simulink model "SCR_Injector_ON_Off"  (R2019a)
settings: Solver=FixedStepAuto  StartTime=0.0  StopTime=100  FixedStep=0.1  RelTol=1e-3
libraries: simulink x4
settings Model: DataDictionary=SCR_Injector_ON_Off_DD.sldd  Creator=Kore  LastModifiedBy=Kore
settings ConfigComp: DVModelCoverageObjectives=MCDC  DVTestSuiteOptimization=Auto  DVDetectDeadLogic=on  DVDetectActiveLogic=on  DVDetectOutOfBounds=on  DVSaveHarnessModel=on  DVSaveReport=on  DVRebuildModelRepresentation=Always

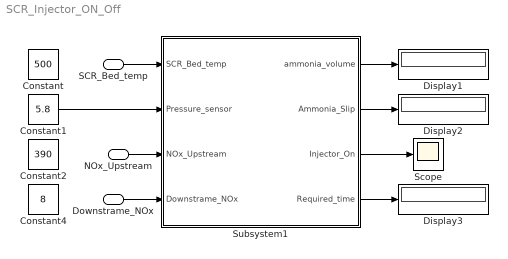
== system SCR_Injector_ON_Off ==
  NOx_Upstream : Inport
  Downstrame_NOx : Inport  Port=2
  SCR_Bed_temp : Inport  Port=3
  Constant : Constant  Value=500
  Constant1 : Constant  Value=5.8
  Constant2 : Constant  Value=390
  Constant4 : Constant  Value=8
  Display1 : Display
  Display2 : Display
  Display3 : Display
  Scope : Scope
  Subsystem1 : Subsystem
  wires:
  Subsystem1/2(Ammonia_Slip) -> Display2/1
  Subsystem1/1(ammonia_volume) -> Display1/1
  Subsystem1/3(Injector_On) -> Scope/1
  Subsystem1/4(Required_time) -> Display3/1
  Downstrame_NOx/1 -> Subsystem1/4(Downstrame_NOx)
  NOx_Upstream/1 -> Subsystem1/3(NOx_Upstream)
  SCR_Bed_temp/1 -> Subsystem1/1(SCR_Bed_temp)
  Constant1/1 -> Subsystem1/2(Pressure_sensor)

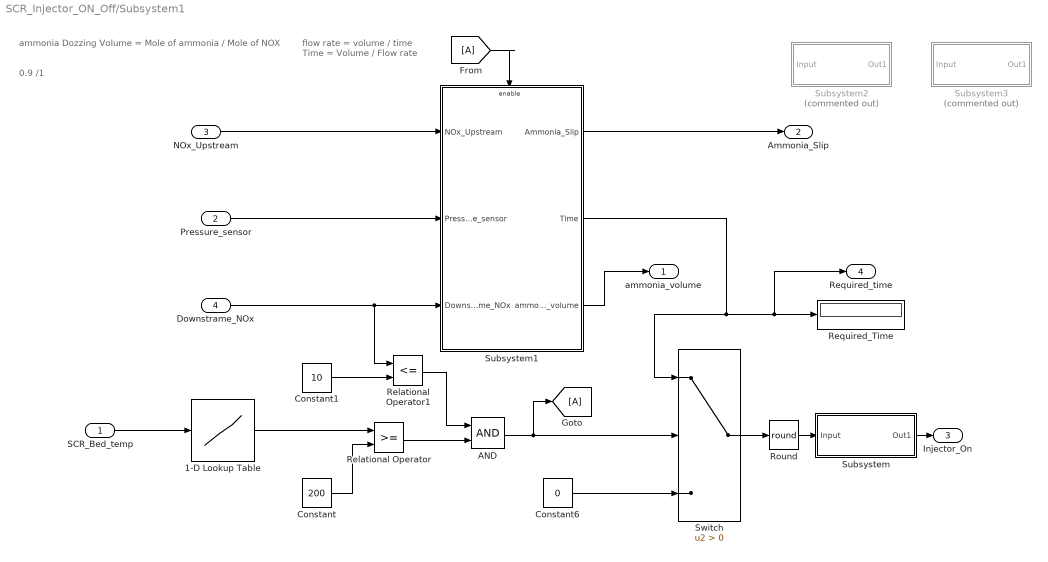
== system SCR_Injector_ON_Off/Subsystem1 ==
  note: 0.9 /1
  note: ammonia Dozzing Volume = Mole of ammonia / Mole of NOX
  note: flow rate = volume / time
      |
      | Time = Volume / Flow rate
  SCR_Bed_temp : Inport
  Pressure_sensor : Inport  Port=2
  NOx_Upstream : Inport  Port=3
  Downstrame_NOx : Inport  Port=4
  1-D Lookup Table : Lookup_n-D  NumberOfTableDimensions=1  BreakpointsForDimension1=[1:10:650]  BreakpointsForDimension2=[1:1:500]  Table=[1:10:650]  InternalRulePriority=Speed  RndMeth=Simplest  InputSameDT=on
  AND : Logic  AllPortsSameDT=off  OutDataTypeStr=boolean
  Constant : Constant  Value=200
  Constant1 : Constant  Value=10
  Constant6 : Constant  Value=0
  Relational Operator : RelationalOperator  OutDataTypeStr=boolean  RndMeth=Simplest
  Relational Operator1 : RelationalOperator  Operator=<=  OutDataTypeStr=boolean  RndMeth=Simplest
  Required_Time : Display
  Round : Rounding  Operator=round
  Subsystem : Subsystem
  Subsystem1 : Subsystem
  Subsystem2 : Subsystem  Commented=on
  Subsystem3 : Subsystem  Commented=on
  Switch : Switch  Criteria=u2 > Threshold
  ammonia_volume : Outport
  Ammonia_Slip : Outport  Port=2
  Injector_On : Outport  Port=3
  Required_time : Outport  Port=4
  wires:
  Constant/1 -> Relational Operator/2
  SCR_Bed_temp/1 -> 1-D Lookup Table/1
  1-D Lookup Table/1 -> Relational Operator/1
  Constant6/1 -> Switch/3
  Switch/1 -> Round/1
  Subsystem1/2(Time) -> Switch/1, Required_time/1, Required_Time/1
  NOx_Upstream/1 -> Subsystem1/1(NOx_Upstream)
  Pressure_sensor/1 -> Subsystem1/2(Pressure_sensor)
  Subsystem1/1(Ammonia_Slip) -> Ammonia_Slip/1
  Downstrame_NOx/1 -> Relational Operator1/1, Subsystem1/3(Downstrame_NOx)
  [A] -> Subsystem1/Enable
  Subsystem/1(Out1) -> Injector_On/1
  Round/1 -> Subsystem/1(Input)
  Relational Operator/1 -> AND/2
  AND/1 -> [A], Switch/2
  Relational Operator1/1 -> AND/1
  Constant1/1 -> Relational Operator1/2
  Subsystem1/3(ammonia_volume) -> ammonia_volume/1

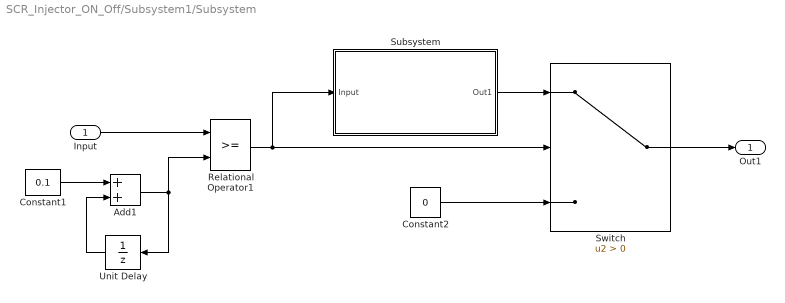
== system SCR_Injector_ON_Off/Subsystem1/Subsystem ==
  Input : Inport
  Add1 : Sum
  Constant1 : Constant  Value=0.1
  Constant2 : Constant  Value=0
  Relational Operator1 : RelationalOperator  OutDataTypeStr=boolean  RndMeth=Simplest
  Subsystem : Subsystem
  Switch : Switch  Criteria=u2 > Threshold
  Unit Delay : UnitDelay  SampleTime=-1  HasFrameUpgradeWarning=on
  Out1 : Outport
  wires:
  Constant2/1 -> Switch/3
  Unit Delay/1 -> Add1/2
  Constant1/1 -> Add1/1
  Add1/1 -> Unit Delay/1, Relational Operator1/2
  Subsystem/1(Out1) -> Switch/1
  Input/1 -> Relational Operator1/1
  Switch/1 -> Out1/1
  Relational Operator1/1 -> Switch/2, Subsystem/1(Input)

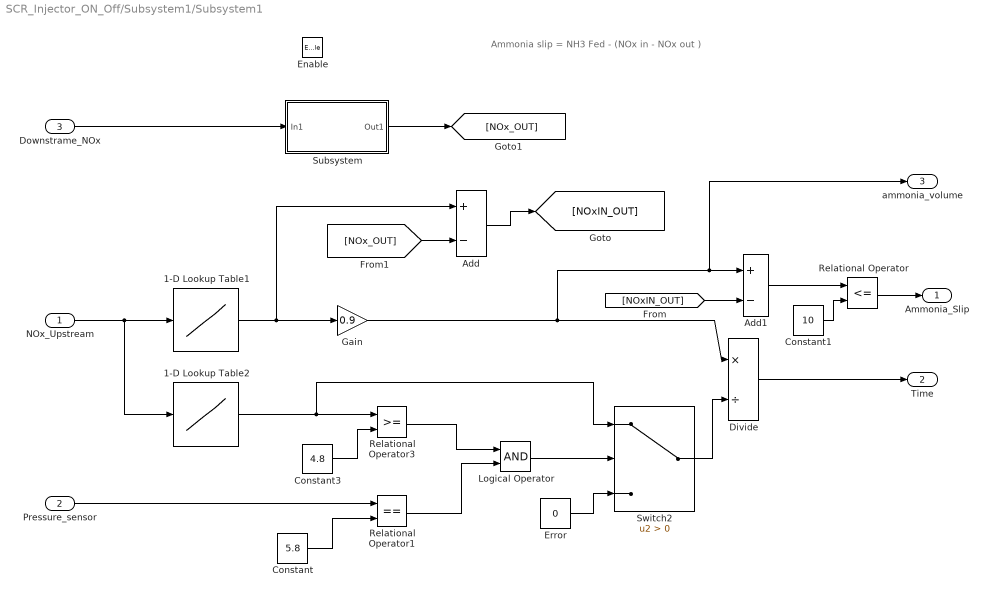
== system SCR_Injector_ON_Off/Subsystem1/Subsystem1 ==
  note: Ammonia slip = NH3 Fed - (NOx in - NOx out )
  NOx_Upstream : Inport
  Pressure_sensor : Inport  Port=2
  Downstrame_NOx : Inport  Port=3
  Enable : EnablePort  StatesWhenEnabling=reset
  1-D Lookup Table1 : Lookup_n-D  NumberOfTableDimensions=1  BreakpointsForDimension1=[1:5:650]  BreakpointsForDimension2=[1:1:500]  Table=[1:5:650]  InternalRulePriority=Speed  RndMeth=Simplest  InputSameDT=on
  1-D Lookup Table2 : Lookup_n-D  NumberOfTableDimensions=1  BreakpointsForDimension1=|  BreakpointsForDimension2=[1:1:500]  Table=|  InternalRulePriority=Speed  RndMeth=Simplest  InputSameDT=on
      BreakpointsForDimension1=|
      | [10
      | 70
      | 77.6
      | 80.4
      | 86.4
      | 99.6
      | 108
      | 117.6
      | 127.2
      | 136.8
      | 149.3
      | 158.3
      | 163.3
      | 168.3
      | 175.3
      | 181.5
      | 187.7
      | 193.9
      | 200.1
      | 206.3
      | 212.85
      | 223.5
      | 233.15
      | 242.8
      | 255.45
      | 264.9
      | 275.35
      | 285.8
      | 296.25
      | 306.7
      | 317.15
      | 327.6
      | 338.05
      | 348.5
      | 358.95
      | 369.4
      | 379.85
      | 390.3
      | 400.75
      | 411.2
      | 421.65
      | 432.1
      | 442.55
      | 453
      | 463.45
      | 473.9
      | 484.35
      | 494.8
      | 505.25
      | 515.7
      | 526.15
      | 536.6
      | 547.05
      | 557.5]
      Table=|
      | [4
      | 4
      | 4
      | 4
      | 4
      | 4
      | 4
      | 4
      | 4
      | 4.8
      | 4.8
      | 4.8
      | 4.8
      | 4.8
      | 4.8
      | 4.8
      | 4.8
      | 4.8
      | 4.8
      | 4.8
      | 4.8
      | 5.8
      | 6.4
      | 7.3
      | 8.1
      | 8.9
      | 9.7
      | 10.5
      | 11.3
      | 12.1
      | 12.9
      | 13.7
      | 14.5
      | 15.3
      | 16.1
      | 16.9
      | 17.7
      | 18.5
      | 19.3
      | 20.1
      | 20.9
      | 21.7
      | 22.5
      | 23.3
      | 24.1
      | 24.9
      | 25.7
      | 26.5
      | 27.3
      | 28.1
      | 28.9
      | 29.7
      | 30.0
      | 30.0
      | ]
  Add : Sum  Inputs=+-
  Add1 : Sum  Inputs=+-
  Constant : Constant  Value=5.8
  Constant1 : Constant  Value=10
  Constant3 : Constant  Value=4.8
  Divide : Product  Inputs=*/
  Error : Constant  Value=0
  Gain : Gain  Gain=0.9
  Logical Operator : Logic  AllPortsSameDT=off  OutDataTypeStr=boolean
  Relational Operator : RelationalOperator  Operator=<=  OutDataTypeStr=boolean  RndMeth=Simplest
  Relational Operator1 : RelationalOperator  Operator===  OutDataTypeStr=boolean  RndMeth=Simplest
  Relational Operator3 : RelationalOperator  OutDataTypeStr=boolean  RndMeth=Simplest
  Subsystem : Subsystem
  Switch2 : Switch  Criteria=u2 > Threshold
  Ammonia_Slip : Outport
  Time : Outport  Port=2
  ammonia_volume : Outport  Port=3
  wires:
  Pressure_sensor/1 -> Relational Operator1/1
  Add/1 -> [NOxIN_OUT]
  [NOx_OUT] -> Add/2
  Relational Operator1/1 -> Logical Operator/2
  Constant/1 -> Relational Operator1/2
  1-D Lookup Table1/1 -> Gain/1, Add/1
  Divide/1 -> Time/1
  Constant3/1 -> Relational Operator3/2
  Relational Operator3/1 -> Logical Operator/1
  Error/1 -> Switch2/3
  Switch2/1 -> Divide/2
  Logical Operator/1 -> Switch2/2
  [NOxIN_OUT] -> Add1/2
  Add1/1 -> Relational Operator/1
  Subsystem/1(Out1) -> [NOx_OUT]
  Downstrame_NOx/1 -> Subsystem/1(In1)
  1-D Lookup Table2/1 -> Switch2/1, Relational Operator3/1
  NOx_Upstream/1 -> 1-D Lookup Table2/1, 1-D Lookup Table1/1
  Constant1/1 -> Relational Operator/2
  Relational Operator/1 -> Ammonia_Slip/1
  Gain/1 -> Divide/1, ammonia_volume/1, Add1/1

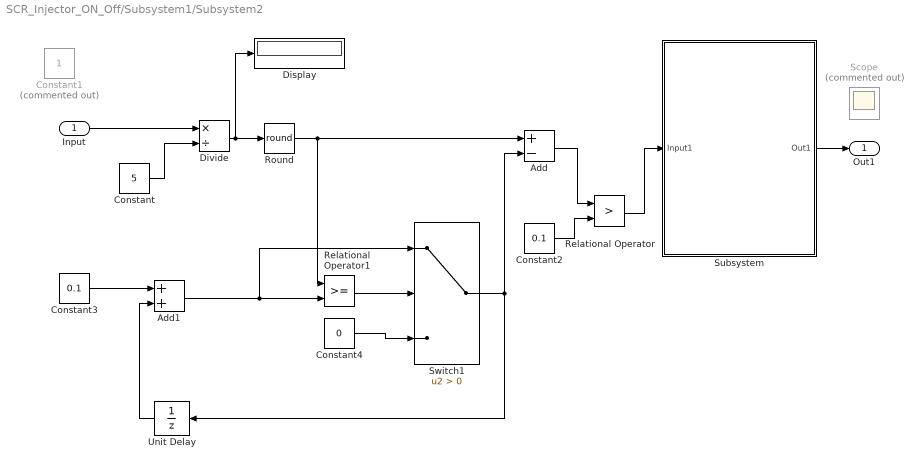
== system SCR_Injector_ON_Off/Subsystem1/Subsystem2 ==
  Input : Inport
  Add : Sum  Inputs=+-
  Add1 : Sum
  Constant : Constant  Value=5
  Constant1 : Constant  Commented=on
  Constant2 : Constant  Value=0.1
  Constant3 : Constant  Value=0.1
  Constant4 : Constant  Value=0
  Display : Display
  Divide : Product  Inputs=*/
  Relational Operator : RelationalOperator  Operator=>  OutDataTypeStr=boolean  RndMeth=Simplest
  Relational Operator1 : RelationalOperator  OutDataTypeStr=boolean  RndMeth=Simplest
  Round : Rounding  Operator=round
  Scope : Scope  Commented=on
  Subsystem : Subsystem
  Switch1 : Switch  Criteria=u2 > Threshold
  Unit Delay : UnitDelay  SampleTime=-1  HasFrameUpgradeWarning=on
  Out1 : Outport
  wires:
  Constant/1 -> Divide/2
  Divide/1 -> Round/1, Display/1
  Input/1 -> Divide/1
  Round/1 -> Relational Operator1/1, Add/1
  Constant4/1 -> Switch1/3
  Switch1/1 -> Add/2, Unit Delay/1
  Constant3/1 -> Add1/1
  Relational Operator1/1 -> Switch1/2
  Add1/1 -> Switch1/1, Relational Operator1/2
  Unit Delay/1 -> Add1/2
  Subsystem/1(Out1) -> Out1/1
  Add/1 -> Relational Operator/1
  Relational Operator/1 -> Subsystem/1(Input1)
  Constant2/1 -> Relational Operator/2

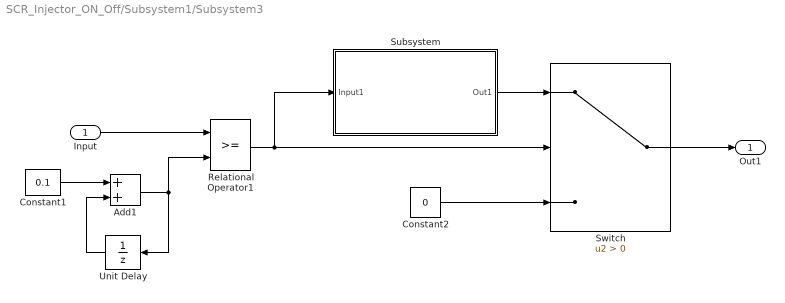
== system SCR_Injector_ON_Off/Subsystem1/Subsystem3 ==
  Input : Inport
  Add1 : Sum
  Constant1 : Constant  Value=0.1
  Constant2 : Constant  Value=0
  Relational Operator1 : RelationalOperator  OutDataTypeStr=boolean  RndMeth=Simplest
  Subsystem : Subsystem
  Switch : Switch  Criteria=u2 > Threshold
  Unit Delay : UnitDelay  SampleTime=-1  HasFrameUpgradeWarning=on
  Out1 : Outport
  wires:
  Relational Operator1/1 -> Switch/2, Subsystem/1(Input1)
  Switch/1 -> Out1/1
  Input/1 -> Relational Operator1/1
  Subsystem/1(Out1) -> Switch/1
  Add1/1 -> Relational Operator1/2, Unit Delay/1
  Constant1/1 -> Add1/1
  Unit Delay/1 -> Add1/2
  Constant2/1 -> Switch/3

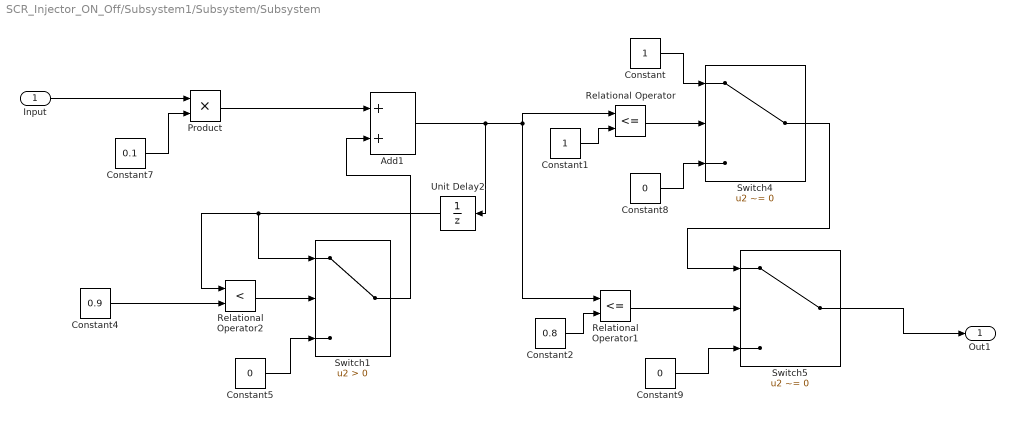
== system SCR_Injector_ON_Off/Subsystem1/Subsystem/Subsystem ==
  Input : Inport
  Add1 : Sum
  Constant : Constant
  Constant1 : Constant
  Constant2 : Constant  Value=0.8
  Constant4 : Constant  Value=0.9
  Constant5 : Constant  Value=0
  Constant7 : Constant  Value=0.1
  Constant8 : Constant  Value=0
  Constant9 : Constant  Value=0
  Product : Product
  Relational Operator : RelationalOperator  Operator=<=  OutDataTypeStr=boolean  RndMeth=Simplest
  Relational Operator1 : RelationalOperator  Operator=<=  OutDataTypeStr=boolean  RndMeth=Simplest
  Relational Operator2 : RelationalOperator  Operator=<  OutDataTypeStr=boolean  RndMeth=Simplest
  Switch1 : Switch  Criteria=u2 > Threshold
  Switch4 : Switch  Criteria=u2 ~= 0
  Switch5 : Switch  Criteria=u2 ~= 0
  Unit Delay2 : UnitDelay  SampleTime=-1  HasFrameUpgradeWarning=on
  Out1 : Outport
  wires:
  Switch5/1 -> Out1/1
  Constant5/1 -> Switch1/3
  Switch1/1 -> Add1/2
  Switch4/1 -> Switch5/1
  Constant9/1 -> Switch5/3
  Relational Operator2/1 -> Switch1/2
  Constant8/1 -> Switch4/3
  Unit Delay2/1 -> Switch1/1, Relational Operator2/1
  Constant4/1 -> Relational Operator2/2
  Constant/1 -> Switch4/1
  Constant7/1 -> Product/2
  Product/1 -> Add1/1
  Input/1 -> Product/1
  Constant1/1 -> Relational Operator/2
  Relational Operator/1 -> Switch4/2
  Constant2/1 -> Relational Operator1/2
  Add1/1 -> Unit Delay2/1, Relational Operator/1, Relational Operator1/1
  Relational Operator1/1 -> Switch5/2

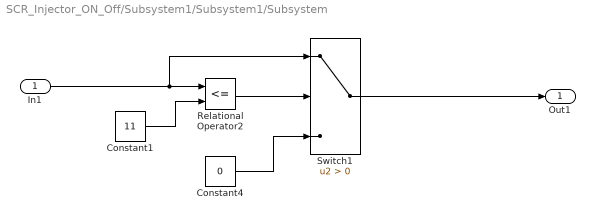
== system SCR_Injector_ON_Off/Subsystem1/Subsystem1/Subsystem ==
  In1 : Inport
  Constant1 : Constant  Value=11
  Constant4 : Constant  Value=0
  Relational Operator2 : RelationalOperator  Operator=<=  OutDataTypeStr=boolean  RndMeth=Simplest
  Switch1 : Switch  Criteria=u2 > Threshold
  Out1 : Outport
  wires:
  Relational Operator2/1 -> Switch1/2
  Switch1/1 -> Out1/1
  Constant1/1 -> Relational Operator2/2
  In1/1 -> Switch1/1, Relational Operator2/1
  Constant4/1 -> Switch1/3

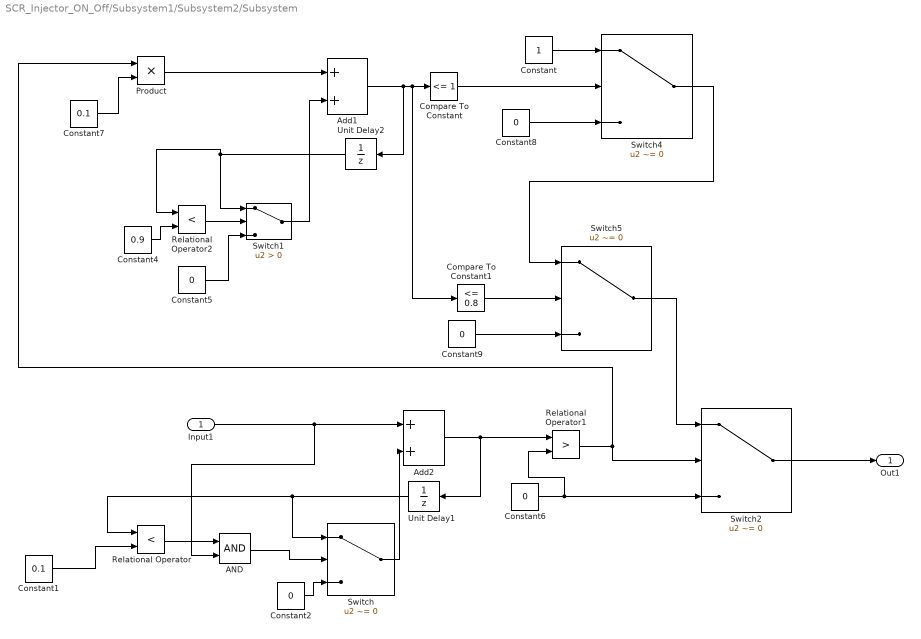
== system SCR_Injector_ON_Off/Subsystem1/Subsystem2/Subsystem ==
  Input1 : Inport
  AND : Logic  AllPortsSameDT=off  OutDataTypeStr=boolean
  Add1 : Sum
  Add2 : Sum
  Compare To Constant : simulink/Logic and Bit Operations/Compare To Constant  relop=<=  const=1  OutDataTypeStr=boolean
  Compare To Constant1 : simulink/Logic and Bit Operations/Compare To Constant  relop=<=  const=0.8  OutDataTypeStr=boolean
  Constant : Constant
  Constant1 : Constant  Value=0.1
  Constant{2,5..6,8..9} (5 alike) : Constant  Value=0
  Constant4 : Constant  Value=0.9
  Constant7 : Constant  Value=0.1
  Product : Product
  Relational Operator : RelationalOperator  Operator=<  OutDataTypeStr=boolean  RndMeth=Simplest
  Relational Operator1 : RelationalOperator  Operator=>  OutDataTypeStr=boolean  RndMeth=Simplest
  Relational Operator2 : RelationalOperator  Operator=<  OutDataTypeStr=boolean  RndMeth=Simplest
  Switch{,2,4..5} (4 alike) : Switch  Criteria=u2 ~= 0
  Switch1 : Switch  Criteria=u2 > Threshold
  Unit Delay1 : UnitDelay  SampleTime=-1  HasFrameUpgradeWarning=on
  Unit Delay2 : UnitDelay  SampleTime=-1  HasFrameUpgradeWarning=on
  Out1 : Outport
  wires:
  Switch/1 -> Add2/2
  Relational Operator/1 -> AND/1
  Constant1/1 -> Relational Operator/2
  Constant2/1 -> Switch/3
  Constant6/1 -> Relational Operator1/2, Switch2/3
  Input1/1 -> AND/2, Add2/1
  Unit Delay1/1 -> Switch/1, Relational Operator/1
  Relational Operator1/1 -> Product/1, Switch2/2
  Add2/1 -> Unit Delay1/1, Relational Operator1/1
  Switch5/1 -> Switch2/1
  Switch2/1 -> Out1/1
  Constant5/1 -> Switch1/3
  Switch1/1 -> Add1/2
  Switch4/1 -> Switch5/1
  Compare To Constant/1 -> Switch4/2
  Compare To Constant1/1 -> Switch5/2
  Constant9/1 -> Switch5/3
  Relational Operator2/1 -> Switch1/2
  Constant8/1 -> Switch4/3
  Unit Delay2/1 -> Relational Operator2/1, Switch1/1
  Constant4/1 -> Relational Operator2/2
  Constant/1 -> Switch4/1
  Add1/1 -> Unit Delay2/1, Compare To Constant1/1, Compare To Constant/1
  Constant7/1 -> Product/2
  Product/1 -> Add1/1
  AND/1 -> Switch/2

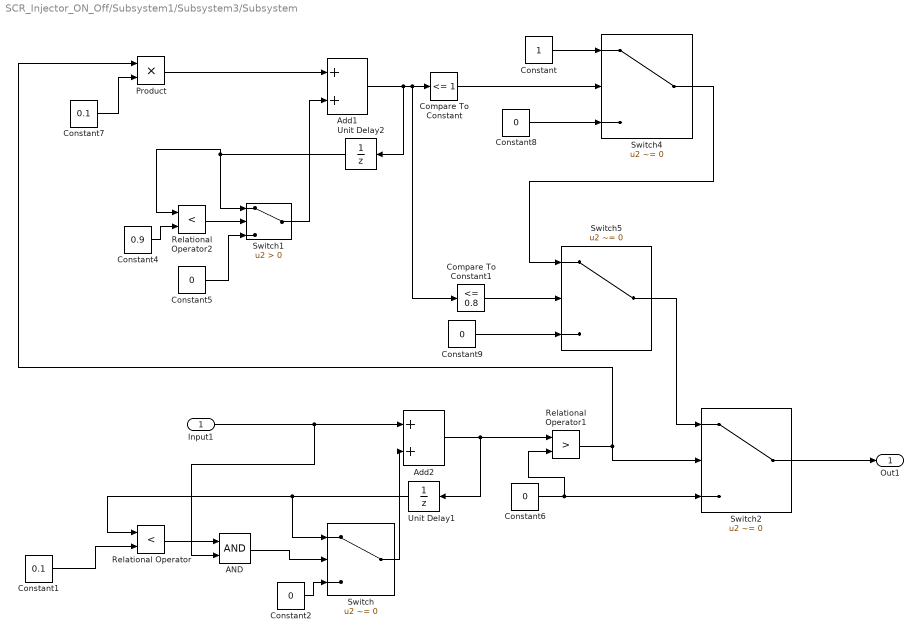
== system SCR_Injector_ON_Off/Subsystem1/Subsystem3/Subsystem ==
  Input1 : Inport
  AND : Logic  AllPortsSameDT=off  OutDataTypeStr=boolean
  Add1 : Sum
  Add2 : Sum
  Compare To Constant : simulink/Logic and Bit Operations/Compare To Constant  relop=<=  const=1  OutDataTypeStr=boolean
  Compare To Constant1 : simulink/Logic and Bit Operations/Compare To Constant  relop=<=  const=0.8  OutDataTypeStr=boolean
  Constant : Constant
  Constant1 : Constant  Value=0.1
  Constant{2,5..6,8..9} (5 alike) : Constant  Value=0
  Constant4 : Constant  Value=0.9
  Constant7 : Constant  Value=0.1
  Product : Product
  Relational Operator : RelationalOperator  Operator=<  OutDataTypeStr=boolean  RndMeth=Simplest
  Relational Operator1 : RelationalOperator  Operator=>  OutDataTypeStr=boolean  RndMeth=Simplest
  Relational Operator2 : RelationalOperator  Operator=<  OutDataTypeStr=boolean  RndMeth=Simplest
  Switch{,2,4..5} (4 alike) : Switch  Criteria=u2 ~= 0
  Switch1 : Switch  Criteria=u2 > Threshold
  Unit Delay1 : UnitDelay  SampleTime=-1  HasFrameUpgradeWarning=on
  Unit Delay2 : UnitDelay  SampleTime=-1  HasFrameUpgradeWarning=on
  Out1 : Outport
  wires:
  AND/1 -> Switch/2
  Product/1 -> Add1/1
  Constant7/1 -> Product/2
  Add1/1 -> Compare To Constant/1, Compare To Constant1/1, Unit Delay2/1
  Constant/1 -> Switch4/1
  Constant4/1 -> Relational Operator2/2
  Unit Delay2/1 -> Switch1/1, Relational Operator2/1
  Constant8/1 -> Switch4/3
  Relational Operator2/1 -> Switch1/2
  Constant9/1 -> Switch5/3
  Compare To Constant1/1 -> Switch5/2
  Compare To Constant/1 -> Switch4/2
  Switch4/1 -> Switch5/1
  Switch1/1 -> Add1/2
  Constant5/1 -> Switch1/3
  Switch2/1 -> Out1/1
  Switch5/1 -> Switch2/1
  Add2/1 -> Relational Operator1/1, Unit Delay1/1
  Relational Operator1/1 -> Switch2/2, Product/1
  Unit Delay1/1 -> Relational Operator/1, Switch/1
  Input1/1 -> Add2/1, AND/2
  Constant6/1 -> Switch2/3, Relational Operator1/2
  Constant2/1 -> Switch/3
  Constant1/1 -> Relational Operator/2
  Relational Operator/1 -> AND/1
  Switch/1 -> Add2/2
